simulink model "SOC_Estimation_using_kalman_filter"  (R2025b)
settings: Solver=VariableStepAuto  StartTime=0.0  StopTime=500  RelTol=1e-3
settings Model: Creator=91934  LastModifiedBy=91934

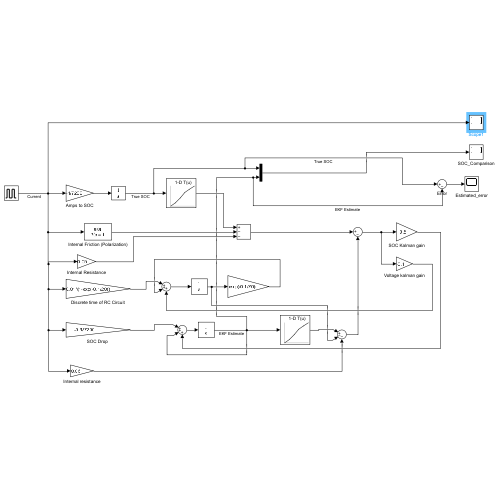
[thumbnail: Simulink's stored preview of the top-level diagram]
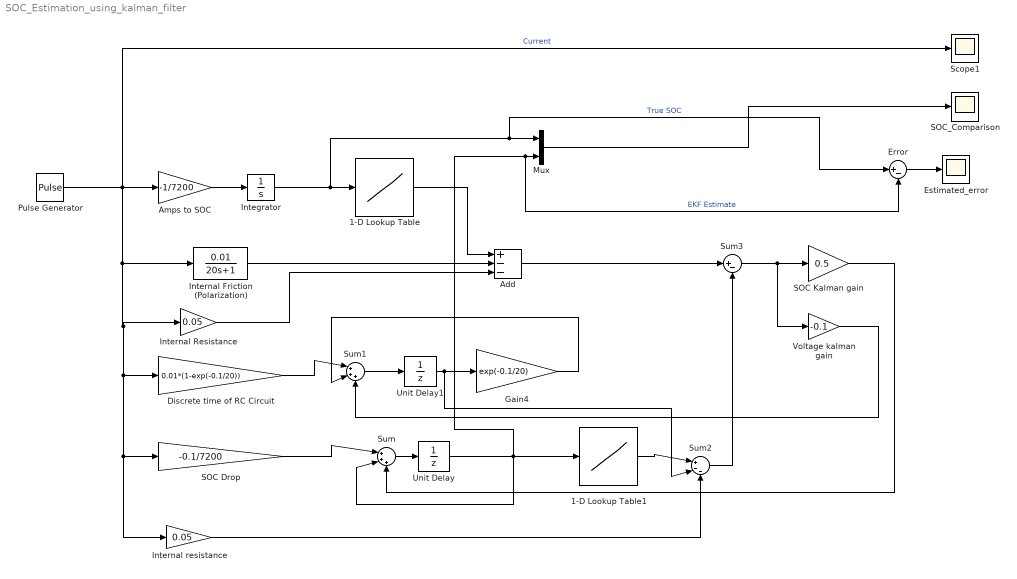
== system SOC_Estimation_using_kalman_filter ==
  1-D Lookup Table : Lookup_n-D  NumberOfTableDimensions=1  BreakpointsForDimension1=[0, 0.2, 0.4, 0.6, 0.8, 1]  Table=[3, 3.2, 3.5, 3.8, 4, 4.2]  InternalRulePriority=Speed  RndMeth=Simplest
  1-D Lookup Table1 : Lookup_n-D  NumberOfTableDimensions=1  BreakpointsForDimension1=[0, 0.2, 0.4, 0.6, 0.8, 1]  Table=[3, 3.2, 3.5, 3.8, 4, 4.2]  InternalRulePriority=Speed  RndMeth=Simplest
  Add : Sum  Inputs=+--
  Amps to SOC : Gain  Gain=-1/7200
  Discrete time of RC Circuit : Gain  Gain=0.01*(1-exp(-0.1/20))
  Error : Sum  Inputs=|+-
  Estimated_error : Scope
      settings: ActiveDisplayYMinimum=0.0049382015138333124  ActiveDisplayYMaximum=0.555006866498463
  Gain4 : Gain  Gain=exp(-0.1/20)
  Integrator : Integrator  InitialCondition=1
  Internal Friction (Polarization) : TransferFcn  Numerator=[0.01]  Denominator=[20 1]
  Internal Resistance : Gain  Gain=0.05
  Internal resistance : Gain  Gain=0.05
  Mux : Mux  Inputs=2
  Pulse Generator : DiscretePulseGenerator  PulseType=Time based  Amplitude=2  Period=100  PulseWidth=50
  "SOC Drop " : Gain  Gain=-0.1/7200
  SOC Kalman gain : Gain  Gain=0.5
  SOC_Comparison : Scope
      settings: ActiveDisplayYMinimum=0.4375  ActiveDisplayYMaximum=1.0625
  Scope1 : Scope
      settings: ActiveDisplayYMinimum=-0.24999999999999994  ActiveDisplayYMaximum=2.25  DataLoggingVariableName=ScopeData2
  Sum : Sum  Inputs=|+++
  Sum1 : Sum  Inputs=|+++
  Sum2 : Sum  Inputs=|+--
  Sum3 : Sum  Inputs=|+-
  Unit Delay : UnitDelay  InitialCondition=0.5  SampleTime=-1  HasFrameUpgradeWarning=on
  Unit Delay1 : UnitDelay  SampleTime=-1  HasFrameUpgradeWarning=on
  Voltage kalman gain : Gain  Gain=-0.1
  wires:
  Amps to SOC/1 -> Integrator/1
  Pulse Generator/1 -> Scope1/1, Internal resistance/1, "SOC Drop "/1, Discrete time of RC Circuit/1, Internal Resistance/1, Internal Friction (Polarization)/1, Amps to SOC/1  "Current"
  Integrator/1 -> Error/1, Mux/1, 1-D Lookup Table/1  "True SOC"
  1-D Lookup Table/1 -> Add/1
  Internal Friction (Polarization)/1 -> Add/2
  Internal Resistance/1 -> Add/3
  "SOC Drop "/1 -> Sum/1
  Sum/1 -> Unit Delay/1
  Unit Delay/1 -> Error/2, Mux/2, Sum/2, 1-D Lookup Table1/1  "EKF Estimate"
  Unit Delay1/1 -> Sum2/2, Gain4/1
  Sum1/1 -> Unit Delay1/1
  1-D Lookup Table1/1 -> Sum2/1
  Internal resistance/1 -> Sum2/3
  Add/1 -> Sum3/1
  Sum2/1 -> Sum3/2
  Sum3/1 -> Voltage kalman gain/1, SOC Kalman gain/1
  Discrete time of RC Circuit/1 -> Sum1/1
  Gain4/1 -> Sum1/2
  SOC Kalman gain/1 -> Sum/3
  Voltage kalman gain/1 -> Sum1/3
  Mux/1 -> SOC_Comparison/1
  Error/1 -> Estimated_error/1
